simulink model "Test_Word_Multiplexer_16_to_1_DirSel"  (Simulink 8.7)
settings: Solver=ode45  StartTime=0.0  StopTime=len  RelTol=1e-3
libraries: Miscellaneous x17, commutil2 x1, Word_Multiplexers_Lib x1
settings Model: Creator=N  LastModifiedBy=Jozko Mrkvicka
settings DataIOCC: LimitDataPoints=off
settings DebuggingCC: UnderspecifiedInitializationDetection=Simplified  MergeDetectMultiDrivingBlocksExec=error
settings HardwareCC: ProdBitPerPointer=64  ProdLargestAtomicFloat=Float  ProdIntDivRoundTo=Zero  ProdEndianess=LittleEndian  ProdHWDeviceType=Intel->x86-64 (Windows64)
settings ModelReferenceCC: PropagateSignalLabelsOutOfModel=on

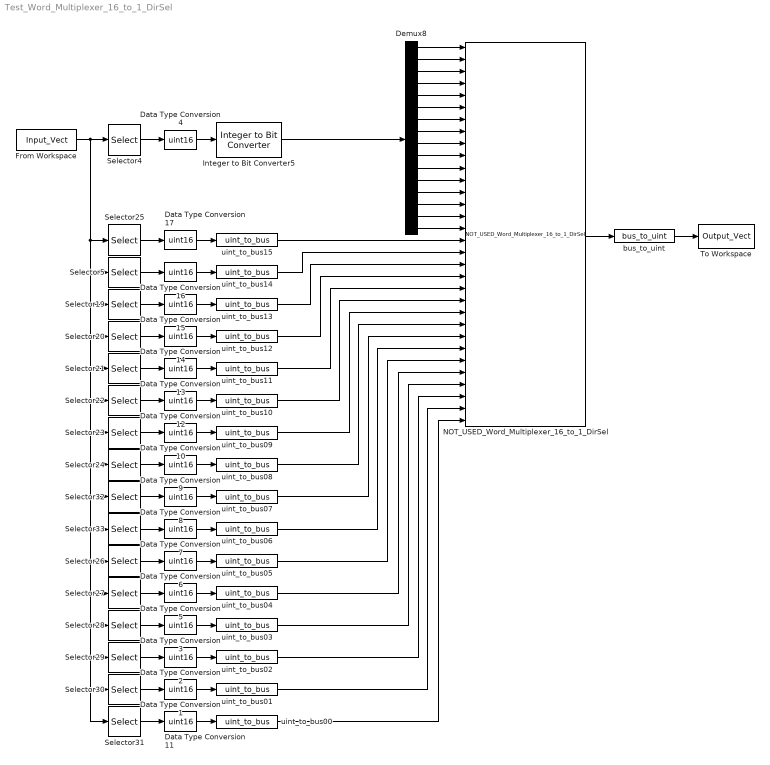
== system Test_Word_Multiplexer_16_to_1_DirSel ==
  Data Type Conversion{1..17} (17 alike) : DataTypeConversion  OutDataTypeStr=uint16
  Demux8 : Demux  Outputs=16
  From Workspace : FromWorkspace  VariableName=Input_Vect  SampleTime=1  Interpolate=off  OutputAfterFinalValue=Holding final value
  Integer to Bit Converter5 : commutil2/Integer to Bit Converter  nbits=16  signedInputValues=Unsigned  bitOrder=MSB first  outDtype=boolean
  NOT_USED_Word_Multiplexer_16_to_1_DirSel : Word_Multiplexers_Lib/Word_Multiplexers_Lib/NOT_USED_Word_Multiplexer_16_to_1_DirSel
  Selector19 : Selector  IndexMode=Zero-based  InputPortWidth=17  IndexOptions=Index vector (dialog)  Indices=3  OutputSizes=1
  Selector20 : Selector  IndexMode=Zero-based  InputPortWidth=17  IndexOptions=Index vector (dialog)  Indices=4  OutputSizes=1
  Selector21 : Selector  IndexMode=Zero-based  InputPortWidth=17  IndexOptions=Index vector (dialog)  Indices=5  OutputSizes=1
  Selector22 : Selector  IndexMode=Zero-based  InputPortWidth=17  IndexOptions=Index vector (dialog)  Indices=6  OutputSizes=1
  Selector23 : Selector  IndexMode=Zero-based  InputPortWidth=17  IndexOptions=Index vector (dialog)  Indices=7  OutputSizes=1
  Selector24 : Selector  IndexMode=Zero-based  InputPortWidth=17  IndexOptions=Index vector (dialog)  Indices=8  OutputSizes=1
  Selector25 : Selector  IndexMode=Zero-based  InputPortWidth=17  IndexOptions=Index vector (dialog)  Indices=1  OutputSizes=1
  Selector26 : Selector  IndexMode=Zero-based  InputPortWidth=17  IndexOptions=Index vector (dialog)  Indices=11  OutputSizes=1
  Selector27 : Selector  IndexMode=Zero-based  InputPortWidth=17  IndexOptions=Index vector (dialog)  Indices=12  OutputSizes=1
  Selector28 : Selector  IndexMode=Zero-based  InputPortWidth=17  IndexOptions=Index vector (dialog)  Indices=13  OutputSizes=1
  Selector29 : Selector  IndexMode=Zero-based  InputPortWidth=17  IndexOptions=Index vector (dialog)  Indices=14  OutputSizes=1
  Selector30 : Selector  IndexMode=Zero-based  InputPortWidth=17  IndexOptions=Index vector (dialog)  Indices=15  OutputSizes=1
  Selector31 : Selector  IndexMode=Zero-based  InputPortWidth=17  IndexOptions=Index vector (dialog)  Indices=16  OutputSizes=1
  Selector32 : Selector  IndexMode=Zero-based  InputPortWidth=17  IndexOptions=Index vector (dialog)  Indices=9  OutputSizes=1
  Selector33 : Selector  IndexMode=Zero-based  InputPortWidth=17  IndexOptions=Index vector (dialog)  Indices=10  OutputSizes=1
  Selector4 : Selector  IndexMode=Zero-based  InputPortWidth=17  SampleTime=1  IndexOptions=Index vector (dialog)  Indices=0  OutputSizes=1
  Selector5 : Selector  IndexMode=Zero-based  InputPortWidth=17  IndexOptions=Index vector (dialog)  Indices=2  OutputSizes=1
  To Workspace : ToWorkspace  VariableName=Output_Vect  SampleTime=1
  bus_to_uint : Miscellaneous/bus_to_uint
  uint_to_bus00 : Miscellaneous/uint_to_bus
  uint_to_bus01 : Miscellaneous/uint_to_bus
  uint_to_bus02 : Miscellaneous/uint_to_bus
  uint_to_bus03 : Miscellaneous/uint_to_bus
  uint_to_bus04 : Miscellaneous/uint_to_bus
  uint_to_bus05 : Miscellaneous/uint_to_bus
  uint_to_bus06 : Miscellaneous/uint_to_bus
  uint_to_bus07 : Miscellaneous/uint_to_bus
  uint_to_bus08 : Miscellaneous/uint_to_bus
  uint_to_bus09 : Miscellaneous/uint_to_bus
  uint_to_bus{10..15} (6 alike) : Miscellaneous/uint_to_bus
  wires:
  Integer to Bit Converter5/1 -> Demux8/1
  NOT_USED_Word_Multiplexer_16_to_1_DirSel/1 -> bus_to_uint/1
  Selector4/1 -> Data Type Conversion4/1
  Data Type Conversion4/1 -> Integer to Bit Converter5/1
  From Workspace/1 -> Selector5/1, Selector19/1, Selector20/1, Selector21/1, Selector22/1, Selector23/1, Selector32/1, Selector33/1, Selector26/1, Selector27/1, Selector28/1, Selector29/1, Selector30/1, Selector31/1, Selector24/1, Selector25/1, Selector4/1
  Selector25/1 -> Data Type Conversion17/1
  Selector5/1 -> Data Type Conversion16/1
  Selector19/1 -> Data Type Conversion15/1
  Selector20/1 -> Data Type Conversion14/1
  Selector21/1 -> Data Type Conversion13/1
  Selector22/1 -> Data Type Conversion12/1
  Selector23/1 -> Data Type Conversion10/1
  Selector24/1 -> Data Type Conversion9/1
  Selector32/1 -> Data Type Conversion8/1
  Selector33/1 -> Data Type Conversion7/1
  Selector26/1 -> Data Type Conversion6/1
  Selector27/1 -> Data Type Conversion5/1
  Selector28/1 -> Data Type Conversion3/1
  Selector29/1 -> Data Type Conversion2/1
  Selector30/1 -> Data Type Conversion1/1
  Selector31/1 -> Data Type Conversion11/1
  Data Type Conversion17/1 -> uint_to_bus15/1
  Data Type Conversion16/1 -> uint_to_bus14/1
  Data Type Conversion15/1 -> uint_to_bus13/1
  Data Type Conversion14/1 -> uint_to_bus12/1
  Data Type Conversion13/1 -> uint_to_bus11/1
  Data Type Conversion12/1 -> uint_to_bus10/1
  Data Type Conversion10/1 -> uint_to_bus09/1
  Data Type Conversion9/1 -> uint_to_bus08/1
  Data Type Conversion8/1 -> uint_to_bus07/1
  Data Type Conversion7/1 -> uint_to_bus06/1
  Data Type Conversion6/1 -> uint_to_bus05/1
  Data Type Conversion5/1 -> uint_to_bus04/1
  Data Type Conversion3/1 -> uint_to_bus03/1
  Data Type Conversion2/1 -> uint_to_bus02/1
  Data Type Conversion1/1 -> uint_to_bus01/1
  Data Type Conversion11/1 -> uint_to_bus00/1
  bus_to_uint/1 -> To Workspace/1
  uint_to_bus00/1 -> NOT_USED_Word_Multiplexer_16_to_1_DirSel/32
  uint_to_bus01/1 -> NOT_USED_Word_Multiplexer_16_to_1_DirSel/31
  uint_to_bus02/1 -> NOT_USED_Word_Multiplexer_16_to_1_DirSel/30
  uint_to_bus03/1 -> NOT_USED_Word_Multiplexer_16_to_1_DirSel/29
  uint_to_bus04/1 -> NOT_USED_Word_Multiplexer_16_to_1_DirSel/28
  uint_to_bus05/1 -> NOT_USED_Word_Multiplexer_16_to_1_DirSel/27
  uint_to_bus06/1 -> NOT_USED_Word_Multiplexer_16_to_1_DirSel/26
  uint_to_bus07/1 -> NOT_USED_Word_Multiplexer_16_to_1_DirSel/25
  uint_to_bus08/1 -> NOT_USED_Word_Multiplexer_16_to_1_DirSel/24
  uint_to_bus09/1 -> NOT_USED_Word_Multiplexer_16_to_1_DirSel/23
  uint_to_bus10/1 -> NOT_USED_Word_Multiplexer_16_to_1_DirSel/22
  uint_to_bus11/1 -> NOT_USED_Word_Multiplexer_16_to_1_DirSel/21
  uint_to_bus12/1 -> NOT_USED_Word_Multiplexer_16_to_1_DirSel/20
  uint_to_bus13/1 -> NOT_USED_Word_Multiplexer_16_to_1_DirSel/19
  uint_to_bus14/1 -> NOT_USED_Word_Multiplexer_16_to_1_DirSel/18
  uint_to_bus15/1 -> NOT_USED_Word_Multiplexer_16_to_1_DirSel/17
  Demux8/1 -> NOT_USED_Word_Multiplexer_16_to_1_DirSel/1
  Demux8/2 -> NOT_USED_Word_Multiplexer_16_to_1_DirSel/2
  Demux8/4 -> NOT_USED_Word_Multiplexer_16_to_1_DirSel/4
  Demux8/3 -> NOT_USED_Word_Multiplexer_16_to_1_DirSel/3
  Demux8/5 -> NOT_USED_Word_Multiplexer_16_to_1_DirSel/5
  Demux8/6 -> NOT_USED_Word_Multiplexer_16_to_1_DirSel/6
  Demux8/7 -> NOT_USED_Word_Multiplexer_16_to_1_DirSel/7
  Demux8/8 -> NOT_USED_Word_Multiplexer_16_to_1_DirSel/8
  Demux8/9 -> NOT_USED_Word_Multiplexer_16_to_1_DirSel/9
  Demux8/10 -> NOT_USED_Word_Multiplexer_16_to_1_DirSel/10
  Demux8/11 -> NOT_USED_Word_Multiplexer_16_to_1_DirSel/11
  Demux8/12 -> NOT_USED_Word_Multiplexer_16_to_1_DirSel/12
  Demux8/13 -> NOT_USED_Word_Multiplexer_16_to_1_DirSel/13
  Demux8/14 -> NOT_USED_Word_Multiplexer_16_to_1_DirSel/14
  Demux8/15 -> NOT_USED_Word_Multiplexer_16_to_1_DirSel/15
  Demux8/16 -> NOT_USED_Word_Multiplexer_16_to_1_DirSel/16
